simulink model "TfExplo"  (R2017b)
settings: Solver=VariableStepAuto  StartTime=0.0  StopTime=10  MaxStep=1e-4  RelTol=1e-3
settings Model: Creator=bikulborthakur  LastModifiedBy=bikulborthakur

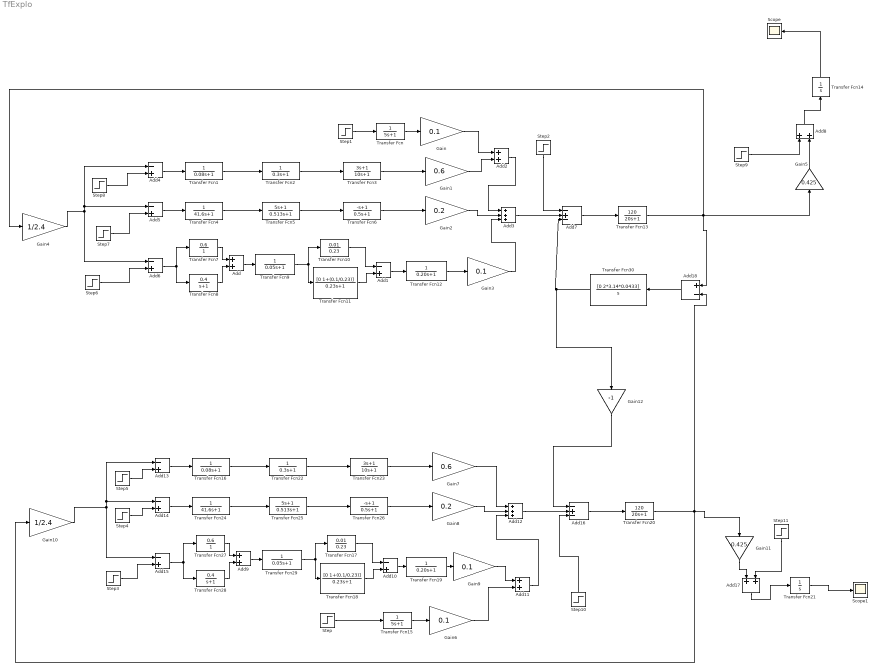
== system TfExplo ==
  Add{,2,8..9,11,17} (6 alike) : Sum
  Add{1,4..6,10,13..15} (8 alike) : Sum  Inputs=-+
  Add12 : Sum  Inputs=+++
  Add16 : Sum  Inputs=-+-
  Add18 : Sum  Inputs=+-
  Add3 : Sum  Inputs=+++
  Add7 : Sum  Inputs=-+-
  Gain{,3,6,9} (4 alike) : Gain  Gain=0.1
  Gain1 : Gain  Gain=0.6
  Gain10 : Gain  Gain=1/2.4
  Gain11 : Gain  Gain=0.425
  Gain12 : Gain  Gain=-1
  Gain2 : Gain  Gain=0.2
  Gain4 : Gain  Gain=1/2.4
  Gain5 : Gain  Gain=0.425
  Gain7 : Gain  Gain=0.6
  Gain8 : Gain  Gain=0.2
  Scope : Scope
  Scope1 : Scope
  Step : Step  Time=0.0001  After=0.01  SampleTime=0.001
  Step1 : Step  Time=0.0001  After=0.01  SampleTime=0.001
  Step10 : Step  Time=0.0001  After=0.001  SampleTime=0.001
  Step{3..9,11} (8 alike) : Step  Time=0.0001  After=10  SampleTime=0.001
  Step2 : Step  Time=0.0001  After=0.01  SampleTime=0.001
  Transfer Fcn : TransferFcn  Denominator=[5 1]
  Transfer Fcn1 : TransferFcn  Denominator=[0.08 1]
  Transfer Fcn10 : TransferFcn  Numerator=[0 0.01]  Denominator=[0 0.23]
  Transfer Fcn11 : TransferFcn  Numerator=[0 1+(0.1/0.23)]  Denominator=[0.23 1]
  Transfer Fcn12 : TransferFcn  Denominator=[0.20 1]
  Transfer Fcn13 : TransferFcn  Numerator=[0 120]  Denominator=[20 1]
  Transfer Fcn14 : TransferFcn  Denominator=[1 0]
  Transfer Fcn15 : TransferFcn  Denominator=[5 1]
  Transfer Fcn16 : TransferFcn  Denominator=[0.08 1]
  Transfer Fcn17 : TransferFcn  Numerator=[0 0.01]  Denominator=[0 0.23]
  Transfer Fcn18 : TransferFcn  Numerator=[0 1+(0.1/0.23)]  Denominator=[0.23 1]
  Transfer Fcn19 : TransferFcn  Denominator=[0.20 1]
  Transfer Fcn2 : TransferFcn  Denominator=[0.3 1]
  Transfer Fcn20 : TransferFcn  Numerator=[0 120]  Denominator=[20 1]
  Transfer Fcn21 : TransferFcn  Denominator=[1 0]
  Transfer Fcn22 : TransferFcn  Denominator=[0.3 1]
  Transfer Fcn23 : TransferFcn  Numerator=[3 1]  Denominator=[10 1]
  Transfer Fcn24 : TransferFcn  Denominator=[41.6 1]
  Transfer Fcn25 : TransferFcn  Numerator=[5 1]  Denominator=[0.513 1]
  Transfer Fcn26 : TransferFcn  Numerator=[-1 1]  Denominator=[0.5 1]
  Transfer Fcn27 : TransferFcn  Numerator=[0 0.6]  Denominator=[0 1]
  Transfer Fcn28 : TransferFcn  Numerator=[0 0.4]  Denominator=[1 1]
  Transfer Fcn29 : TransferFcn  Denominator=[0.05 1]
  Transfer Fcn3 : TransferFcn  Numerator=[3 1]  Denominator=[10 1]
  Transfer Fcn30 : TransferFcn  Numerator=[0 2*3.14*0.0433]  Denominator=[1 0]
  Transfer Fcn4 : TransferFcn  Denominator=[41.6 1]
  Transfer Fcn5 : TransferFcn  Numerator=[5 1]  Denominator=[0.513 1]
  Transfer Fcn6 : TransferFcn  Numerator=[-1 1]  Denominator=[0.5 1]
  Transfer Fcn7 : TransferFcn  Numerator=[0 0.6]  Denominator=[0 1]
  Transfer Fcn8 : TransferFcn  Numerator=[0 0.4]  Denominator=[1 1]
  Transfer Fcn9 : TransferFcn  Denominator=[0.05 1]
  wires:
  Transfer Fcn1/1 -> Transfer Fcn2/1
  Transfer Fcn2/1 -> Transfer Fcn3/1
  Transfer Fcn4/1 -> Transfer Fcn5/1
  Transfer Fcn5/1 -> Transfer Fcn6/1
  Transfer Fcn7/1 -> Add/1
  Transfer Fcn8/1 -> Add/2
  Add/1 -> Transfer Fcn9/1
  Transfer Fcn/1 -> Gain/1
  Transfer Fcn3/1 -> Gain1/1
  Transfer Fcn6/1 -> Gain2/1
  Transfer Fcn12/1 -> Gain3/1
  Add1/1 -> Transfer Fcn12/1
  Transfer Fcn10/1 -> Add1/1
  Transfer Fcn11/1 -> Add1/2
  Transfer Fcn9/1 -> Transfer Fcn11/1, Transfer Fcn10/1
  Gain/1 -> Add2/1
  Gain1/1 -> Add2/2
  Add2/1 -> Add3/1
  Gain2/1 -> Add3/2
  Gain3/1 -> Add3/3
  Add4/1 -> Transfer Fcn1/1
  Add5/1 -> Transfer Fcn4/1
  Add6/1 -> Transfer Fcn8/1, Transfer Fcn7/1
  Gain4/1 -> Add5/1, Add4/1, Add6/1
  Add3/1 -> Add7/2
  Add7/1 -> Transfer Fcn13/1
  Gain5/1 -> Add8/2
  Add8/1 -> Transfer Fcn14/1
  Transfer Fcn13/1 -> Add18/1, Gain4/1, Gain5/1
  Add12/1 -> Add16/2
  Transfer Fcn25/1 -> Transfer Fcn26/1
  Transfer Fcn19/1 -> Gain9/1
  Transfer Fcn22/1 -> Transfer Fcn23/1
  Transfer Fcn16/1 -> Transfer Fcn22/1
  Transfer Fcn29/1 -> Transfer Fcn18/1, Transfer Fcn17/1
  Add15/1 -> Transfer Fcn28/1, Transfer Fcn27/1
  Add14/1 -> Transfer Fcn24/1
  Add16/1 -> Transfer Fcn20/1
  Transfer Fcn27/1 -> Add9/1
  Transfer Fcn28/1 -> Add9/2
  Transfer Fcn18/1 -> Add10/2
  Transfer Fcn20/1 -> Gain10/1, Add18/2, Gain11/1
  Add17/1 -> Transfer Fcn21/1
  Transfer Fcn24/1 -> Transfer Fcn25/1
  Transfer Fcn15/1 -> Gain6/1
  Add10/1 -> Transfer Fcn19/1
  Transfer Fcn26/1 -> Gain8/1
  Add9/1 -> Transfer Fcn29/1
  Transfer Fcn23/1 -> Gain7/1
  Gain8/1 -> Add12/2
  Transfer Fcn17/1 -> Add10/1
  Add13/1 -> Transfer Fcn16/1
  Gain10/1 -> Add14/1, Add13/1, Add15/1
  Add18/1 -> Transfer Fcn30/1
  Gain11/1 -> Add17/1
  Transfer Fcn30/1 -> Gain12/1, Add7/3
  Gain12/1 -> Add16/1
  Gain7/1 -> Add12/1
  Gain9/1 -> Add11/1
  Add11/1 -> Add12/3
  Gain6/1 -> Add11/2
  Step1/1 -> Transfer Fcn/1
  Step2/1 -> Add7/1
  Step/1 -> Transfer Fcn15/1
  Step3/1 -> Add15/2
  Step5/1 -> Add13/2
  Step4/1 -> Add14/2
  Step6/1 -> Add6/2
  Step7/1 -> Add5/2
  Step8/1 -> Add4/2
  Step9/1 -> Add8/1
  Step10/1 -> Add16/3
  Step11/1 -> Add17/2
  Transfer Fcn14/1 -> Scope/1
  Transfer Fcn21/1 -> Scope1/1
